simulink model "move_to_pose"  (R2019b)
settings: Solver=FixedStepAuto  StartTime=0.0  StopTime=inf  FixedStep=sampleTime  RelTol=1e-3
PreLoadFcn:
  | % Simulation parameters
  | load exampleMap
  | sampleTime = 0.05;
  | 
  | % Robot parameters
  | wheelRadius = 0.025;
  | robotRadius = 0.35;
  | 
  | % Lidar parameters
  | sensorOffset = [0,0];
  | scanAngles = linspace(-pi/2,pi/2,9)';
  | maxRange = 5;
undefined symbols (not defined in the file): xy
libraries: mobileRoboticsLib x5, robotalgslib x1, mobileRoboticsTrainingLib x1
settings Model: EnablePacing=on  PacingRate=1000  Creator=scastro  LastModifiedBy=jayas
settings DataIOCC: ReturnWorkspaceOutputs=off
settings DebuggingCC: PregeneratedLibrarySubsystemCodeDiagnostic=none  ArithmeticOperatorsInVariantConditions=warning
settings SFSimCC: SimUseLocalCustomCode=off  CustomCodeUndefinedFunction=UseInterfaceOnly
settings RTWCC: RTWUseLocalCustomCode=off

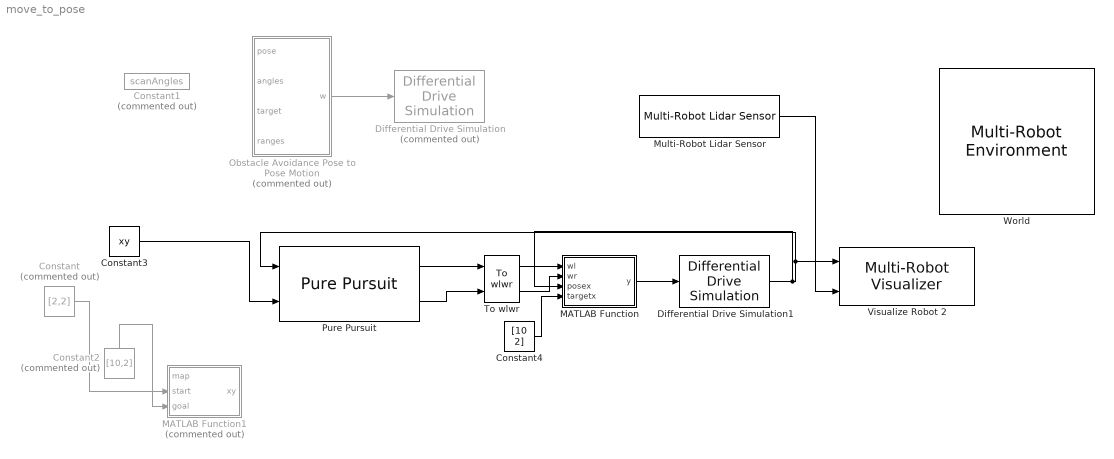
== system move_to_pose ==
  Constant : Constant  Commented=on  Value=[2,2]
  Constant1 : Constant  Commented=on  Value=scanAngles
  Constant2 : Constant  Commented=on  Value=[10,2]
  Constant3 : Constant  Value=xy
  Constant4 : Constant  Value=[10 2]
  Differential Drive Simulation : mobileRoboticsLib/Kinematic Models/Differential Drive/Differential Drive Simulation  Commented=on  wheelRadius=wheelRadius  wheelBase=robotRadius  initX=3  initY=4  initAngle=0  Ts=sampleTime
      settings: SourceProductName=Mobile Robotics Simulation Toolbox
  Differential Drive Simulation1 : mobileRoboticsLib/Kinematic Models/Differential Drive/Differential Drive Simulation  wheelRadius=wheelRadius  wheelBase=robotRadius  initX=2  initY=2  initAngle=0  Ts=sampleTime
      settings: SourceProductName=Mobile Robotics Simulation Toolbox
  MATLAB Function : MATLAB Function  TreatAsAtomicUnit=on
  MATLAB Function1 : MATLAB Function  Commented=on  TreatAsAtomicUnit=on
  Multi-Robot Lidar Sensor : mobileRoboticsLib/Environments/Multi-Robot Lidar Sensor  robotIdx=1  mapName=map  sensorOffset=sensorOffset  scanAngles=scanAngles  maxRange=maxRange
      settings: SourceProductName=Mobile Robotics Simulation Toolbox
  Obstacle Avoidance Pose to Pose Motion : Stateflow chart  Commented=on  TreatAsAtomicUnit=on
  Pure Pursuit : robotalgslib/Pure Pursuit  DesiredLinearVelocity=0.1  MaxAngularVelocity=1  LookaheadDistance=1  TargetDirPort=off  SimulateUsing=Code generation
      settings: SourceProductName=Navigation Toolbox  SourceProductBaseCode=NV
  To wlwr : mobileRoboticsTrainingLib/To wlwr  axleLength=0.1  wheelR=0.05
  Visualize Robot 2 : mobileRoboticsLib/Environments/Multi-Robot Visualizer  idx=1  radius=robotRadius  robotColor=[0 1 1]  showTraj=off  hasLidar=on  sensorOffset=sensorOffset  scanAngles=scanAngles  maxNumScans=0  hasObjDetector=off  objDetectorOffset=[0,0]  objDetectorAngle=0  objDetectorFOV=pi/2  objDetectorMaxRange=5  hasRobotDetector=off  robotDetectorOffset=[0,0]  robotDetectorAngle=0  robotDetectorFOV=pi/3  robotDetectorMaxRange=5  robotDetectorNumDetections=0
      settings: SourceProductName=Mobile Robotics Simulation Toolbox
  World : mobileRoboticsLib/Environments/Multi-Robot Environment  numRobots=1  mapName=map  showWaypoints=off  showObjects=off  objectColors=[1 0 0;0 1 0;0 0 1]  objectMarkers='s'  showRobotIds=on  plotSensorLines=on
      settings: SourceProductName=Mobile Robotics Simulation Toolbox
  wires:
  Obstacle Avoidance Pose to Pose Motion/1(w) -> Differential Drive Simulation/1
  Multi-Robot Lidar Sensor/1 -> Visualize Robot 2/2
  Pure Pursuit/2 -> To wlwr/2
  Pure Pursuit/1 -> To wlwr/1
  To wlwr/1 -> MATLAB Function/1(wl)
  To wlwr/2 -> MATLAB Function/2(wr)
  MATLAB Function/1(y) -> Differential Drive Simulation1/1
  Differential Drive Simulation1/1 -> MATLAB Function/3(posex), Pure Pursuit/1, Visualize Robot 2/1
  Constant/1 -> MATLAB Function1/2(start)
  Constant2/1 -> MATLAB Function1/3(goal)
  Constant3/1 -> Pure Pursuit/2
  Constant4/1 -> MATLAB Function/4(targetx)

== matlab function move_to_pose/MATLAB Function1 ==
  data: map input; start input; xy output; goal input
function xy = fcn(map, start, goal)
    planner = mobileRobotPRM(map);
    xy = findpath(planner, start, goal);
end

== matlab function move_to_pose/MATLAB Function ==
  data: wl input; y output; wr input; posex input; targetx input
function y = fcn(wl, wr, posex, targetx)
    if (abs(posex(1) - targetx(1)) < 0.02 && abs(posex(2) - targetx(2)) < 0.02)
        y = [0 0];
    else
        y = [wl, wr];
    end
end

== stateflow chart move_to_pose/Obstacle Avoidance Pose to Pose Motion ==
  state MainState [parallel]
    en,du:
    validIdx = ~isnan(ranges);
    validRanges = ranges(validIdx);
    validAngles = angles(validIdx);
    settings: executionOrder=1
    state Turn
      en,du:
      avgAngle = mean(validAngles./validRanges);
      state Left
        en, du:
        w = [0;12.5];
      state Right
        en, du:
        w = [12.5;0];
      (default) -> (junction 39)
      (junction 39) -> Left [order 1] : [avgAngle < 0]
      (junction 39) -> (junction 43) [order 2]
      Left -> Right : [after(1,sec) && ...
          | avgAngle > 0]
      Right -> Left : [after(1,sec) && ...
          | avgAngle < 0]
      (junction 43) -> Right
    state AngleCorrection
      en,du:
      x1 = pose(1);
      x2 = target(1);
      y1 = pose(2);
      y2 = target(2);
      targetAngle = get_target_angle(y2-y1, x2-x1);
      w = [0;12.5];
      condition = targetAngle - pose(3);
    state GoStraight1
      en:
      w = [25; 25];
    Turn -> AngleCorrection : [all(validRanges>1)]
    (default) -> AngleCorrection
    GoStraight1 -> Turn : [any(validRanges<=1)]
    AngleCorrection -> GoStraight1 : [condition < 0.05 && condition > -0.05]
  data: y function_input; x function_input; return_value function_output; pose input; angles input; target input; w output; ranges input; validRanges local size=numel(scanAngles); validIdx local; validAngles local size=numel(scanAngles); avgAngle local; targetAngle local; x1 local; x2 local; y1 local; y2 local; condition local
  function return_value = get_target_angle(y, x):
    | function return_value = get_target_angle(y, x)
    |     return_value = atan2(y, x);
    |     if (return_value < 0)
    |         return_value = pi - return_value;
    |     end
    | end
